simulink model "kinematics_2wheel"  (R2019a)
settings: Solver=VariableStepAuto  StartTime=0.0  StopTime=10.0  RelTol=1e-3
settings Model: Creator=chute  LastModifiedBy=chute

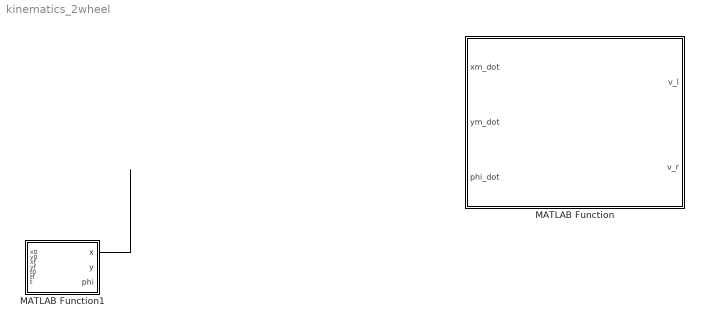
== system kinematics_2wheel ==
  MATLAB Function : MATLAB Function  TreatAsAtomicUnit=on
  MATLAB Function1 : MATLAB Function  TreatAsAtomicUnit=on
  wires:
  MATLAB Function1/1(x) -> ?

== matlab function kinematics_2wheel/MATLAB Function1 ==
  data: x output; y output; phi output; x0 input; y0 input; xf input; yf input; t0 input; tf input; t input
function [x,y,phi] = Trajectory(x0,y0,xf,yf,t0,tf,t)

A=[1 t0 t0^2 t0^3;
   1 tf tf^2 tf^3;
   0 1  2*t0 3*t0^2;
   0 1  2*tf 3*tf^2];
B=[x0,xf,0,0].';
B1 =[y0,yf,0,0].';
X=inv(A)*B;
X1=inv(A)*B1;
a0=X(1);a1=X(2);a2=X(3);a3=X(4);
A0=X(1);A1=X(2);A2=X(3);A3=X(4);
if(t<tf)
    x = a0+a1*(t)+a2*(t.^2)+a3*(t.^3);
    y=A0+A1*(t)+A2*(t.^2)+A3*(t.^3);

y = u;

== matlab function kinematics_2wheel/MATLAB Function ==
  data: xm_dot input; v_l output; ym_dot input; phi_dot input; v_r output
function [v_l,v_r] = fcn(xm_dot,ym_dot,phi_dot)
W=4;
R=0.0325;
J_s=1/R*[cos(phi),sin(phi), W/2;
         cos(phi),sin(phi),-W/2];


y=J_s.*[xm_dot;ym_dot;phi_dot];
v_r=y(1,1);
v_l=y(1,2);
